simulink model "Simulink_Principal_Barbier_Touboul"  (R2020a)
settings: Solver=FixedStepAuto  StartTime=0.0  StopTime=fin  FixedStep=dt  RelTol=1e-4
values from neighbouring files (symbols this model uses):
  A = [teta1;teta2]    [visualisation_trame.m]
  Kd = 20*diag([1 1])    [visualisation_trame.m]
  Kp = 1e3*diag([1 1])    [visualisation_trame.m]
  P = 1e2*diag([1 1])    [visualisation_trame.m]
  S = 1e2*diag([1 1])    [visualisation_trame.m]
  Tau = [T1;T2]    [visualisation_trame.m]
undefined symbols (not defined in the file or in its folder): dyn, dyn2, dyn_mc_1, dyn_mc_2
settings Model: Creator=natha  LastModifiedBy=natha
settings DebuggingCC: ArithmeticOperatorsInVariantConditions=warning
settings SFSimCC: CustomCodeUndefinedFunction=UseInterfaceOnly

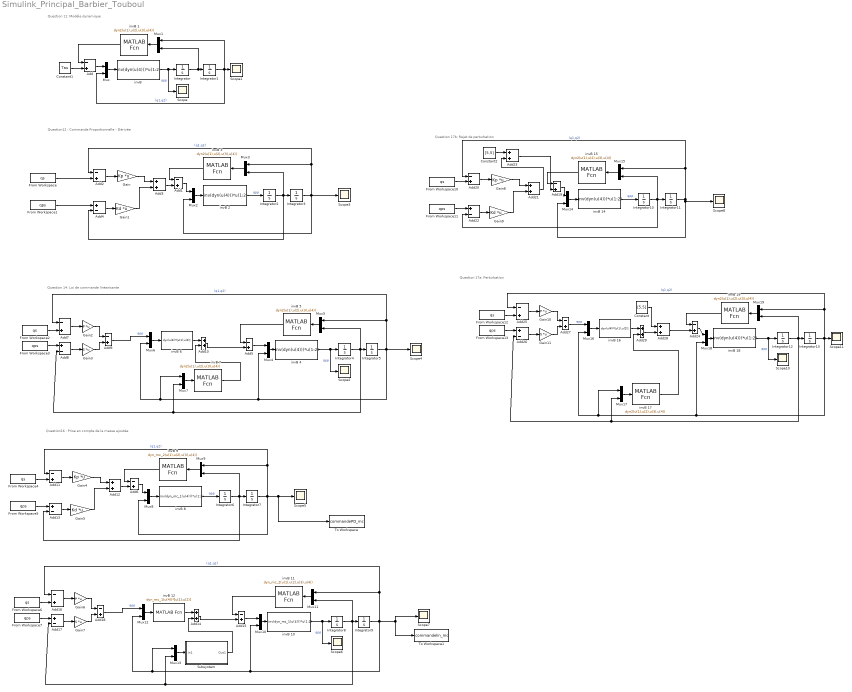
== system Simulink_Principal_Barbier_Touboul ==
  note: Question12 : Commande Proportionnelle - Dérivée
  note: Question 11: Modèle dynamique
  note: Question 14: Loi de commande linéarisante
  note: Question16 : Prise en compte de la masse ajoutée
  note: Question 17b: Rejet de perturbation
  note: Question 17a: Perturbation
  Add{,1..2,5..7,9,11,15..16,18..20,24..25,27} (16 alike) : Sum  Inputs=-+
  Add{3,10,12,14,21,23,28..29} (8 alike) : Sum
  Add{4,8,13,17,22,26} (6 alike) : Sum  Inputs=+-
  Constant : Constant  Value=[5,5]
  Constant1 : Constant  Value=Tau
  Constant2 : Constant  Value=[5,5]
  From Workspace{,2,4,6,10,12} (6 alike) : FromWorkspace  VariableName=qs
  From Workspace{1,3,5,7,11,13} (6 alike) : FromWorkspace  VariableName=qps
  Gain : Gain  Gain=Kp  Multiplication=Matrix(K*u)
  Gain1 : Gain  Gain=Kd  Multiplication=Matrix(K*u)
  Gain10 : Gain  Gain=P  Multiplication=Matrix(K*u)
  Gain11 : Gain  Gain=S  Multiplication=Matrix(K*u)
  Gain2 : Gain  Gain=P  Multiplication=Matrix(K*u)
  Gain3 : Gain  Gain=S  Multiplication=Matrix(K*u)
  Gain4 : Gain  Gain=Kp  Multiplication=Matrix(K*u)
  Gain5 : Gain  Gain=Kd  Multiplication=Matrix(K*u)
  Gain6 : Gain  Gain=P  Multiplication=Matrix(K*u)
  Gain7 : Gain  Gain=S  Multiplication=Matrix(K*u)
  Gain8 : Gain  Gain=Kp  Multiplication=Matrix(K*u)
  Gain9 : Gain  Gain=Kd  Multiplication=Matrix(K*u)
  Integrator{,1..2,4,6,8,10,12} (8 alike) : Integrator
  Integrator{3,5,7,9,11,13} (6 alike) : Integrator  InitialCondition=[A(1,1) A(2,1)]
  Mux{,1..19} (20 alike) : Mux  Inputs=2
  Scope{,1..8,10..11} (11 alike) : Scope
  Subsystem : Subsystem
  To Workspace : ToWorkspace  VariableName=commandePD_mc  SampleTime=-1
  To Workspace1 : ToWorkspace  VariableName=commandelin_mc  SampleTime=-1
  invB {,2,4,14,18} (5 alike) : MATLABFcn  MATLABFcn=inv(dyn(u(4)))*u(1:2)  OutputDimensions=2
      "invB " mask Display: disp('inv(M)*Tau')
      invB 14 mask Display: disp('inv(M)*Tau')
      invB 18 mask Display: disp('inv(M)*(Tau-H)')
      invB 2 mask Display: disp('inv(M)*Tau')
      invB 4 mask Display: disp('inv(M)*(Tau-H)')
  invB {1,3,5,7,15,17,19} (7 alike) : MATLABFcn  MATLABFcn=dyn2(u(1),u(2),u(3),u(4))  OutputDimensions=2
      mask Display: disp('H(q,qp)')
  invB 10 : MATLABFcn  MATLABFcn=inv(dyn_mc_1(u(4)))*u(1:2)  OutputDimensions=2
      mask Display: disp('inv(M)*(Tau-H)')
  invB 11 : MATLABFcn  MATLABFcn=dyn_mc_2(u(1),u(2),u(3),u(4))  OutputDimensions=2
      mask Display: disp('H(q,qp)')
  invB 12 : MATLABFcn  MATLABFcn=dyn_mc_1(u(4))*[u(1);u(2)]  OutputDimensions=2  Output1D=off
      mask Display: disp('M*(epp+qpps)')
  invB 16 : MATLABFcn  MATLABFcn=dyn(u(4))*[u(1);u(2)]  OutputDimensions=2  Output1D=off
      mask Display: disp('M*(epp+qpps)')
  invB 6 : MATLABFcn  MATLABFcn=dyn(u(4))*[u(1);u(2)]  OutputDimensions=2  Output1D=off
      mask Display: disp('M*(epp+qpps)')
  invB 8 : MATLABFcn  MATLABFcn=inv(dyn_mc_1(u(4)))*u(1:2)  OutputDimensions=2
      mask Display: disp('inv(M)*Tau')
  invB 9 : MATLABFcn  MATLABFcn=dyn_mc_2(u(1),u(2),u(3),u(4))  OutputDimensions=2
      mask Display: disp('H(q,qp)')
  wires:
  "invB "/1 -> Scope/1, Integrator/1  "qpp"
  Mux/1 -> "invB "/1
  Constant1/1 -> Add/2
  Integrator/1 -> Mux1/2, Integrator1/1
  Integrator1/1 -> Mux/2, Mux1/1, Scope1/1  "(q1,q2)"
  invB 1/1 -> Add/1
  Add/1 -> Mux/1
  Add1/1 -> Mux2/1
  Mux3/1 -> invB 3/1
  invB 2/1 -> Integrator2/1  "qpp"
  Mux2/1 -> invB 2/1
  invB 3/1 -> Add1/1
  Integrator2/1 -> Add4/2, Mux3/2, Integrator3/1
  Mux1/1 -> invB 1/1
  Add2/1 -> Gain/1
  Add3/1 -> Add1/2
  Gain/1 -> Add3/1
  Add4/1 -> Gain1/1
  Gain1/1 -> Add3/2
  Add10/1 -> Add5/2
  Mux5/1 -> invB 5/1
  invB 7/1 -> Add10/2
  Add9/1 -> Mux6/1  "epp"
  From Workspace2/1 -> Add7/2
  Integrator4/1 -> Add8/2, Mux7/2, Mux5/2, Integrator5/1
  Add7/1 -> Gain2/1
  Add8/1 -> Gain3/1
  Mux7/1 -> invB 7/1
  invB 6/1 -> Add10/1
  Mux4/1 -> invB 4/1
  invB 5/1 -> Add5/1
  Gain2/1 -> Add9/1
  Add5/1 -> Mux4/1
  Gain3/1 -> Add9/2
  invB 4/1 -> Integrator4/1, Scope2/1  "qpp"
  From Workspace3/1 -> Add8/1
  Mux6/1 -> invB 6/1
  From Workspace7/1 -> Add17/1
  Gain7/1 -> Add18/2
  Gain6/1 -> Add18/1
  Integrator9/1 -> Add16/1, Mux11/1, Mux10/2, Mux12/2, Mux13/1, Scope7/1, To Workspace1/1  "(q1,q2)"
  invB 10/1 -> Integrator8/1, Scope6/1  "qpp"
  Add15/1 -> Mux10/1
  invB 11/1 -> Add15/1
  Mux10/1 -> invB 10/1
  invB 12/1 -> Add14/1
  Add16/1 -> Gain6/1
  Mux12/1 -> invB 12/1
  Add17/1 -> Gain7/1
  Integrator8/1 -> Add17/2, Mux13/2, Mux11/2, Integrator9/1
  Add18/1 -> Mux12/1  "epp"
  From Workspace6/1 -> Add16/2
  Mux11/1 -> invB 11/1
  Add14/1 -> Add15/2
  From Workspace4/1 -> Add11/2
  From Workspace5/1 -> Add13/1
  Integrator6/1 -> Add13/2, Mux9/2, Integrator7/1
  Add11/1 -> Gain4/1
  Add13/1 -> Gain5/1
  Add6/1 -> Mux8/1
  invB 8/1 -> Integrator6/1  "qpp"
  Mux8/1 -> invB 8/1
  invB 9/1 -> Add6/1
  Mux9/1 -> invB 9/1
  Integrator7/1 -> Mux8/2, To Workspace/1, Scope5/1, Add11/1, Mux9/1  "(q1,q2)"
  Add12/1 -> Add6/2
  Gain5/1 -> Add12/2
  Gain4/1 -> Add12/1
  From Workspace/1 -> Add2/2
  From Workspace1/1 -> Add4/1
  Integrator10/1 -> Add22/2, Mux15/2, Integrator11/1
  Add23/1 -> Add19/2
  invB 14/1 -> Integrator10/1  "qpp"
  From Workspace10/1 -> Add20/2
  Gain9/1 -> Add21/2
  Mux14/1 -> invB 14/1
  Constant2/1 -> Add23/1
  Integrator3/1 -> Mux2/2, Scope3/1, Add2/1, Mux3/1  "(q1,q2)"
  Add19/1 -> Mux14/1
  Gain8/1 -> Add21/1
  Add22/1 -> Gain9/1
  Integrator11/1 -> Scope8/1, Mux14/2, Add20/1, Mux15/1  "(q1,q2)"
  Add20/1 -> Gain8/1
  Mux15/1 -> invB 15/1
  From Workspace11/1 -> Add22/1
  invB 15/1 -> Add19/1
  Add21/1 -> Add23/2
  From Workspace12/1 -> Add25/2
  Mux18/1 -> invB 18/1
  From Workspace13/1 -> Add26/1
  Integrator13/1 -> Mux16/2, Mux17/1, Mux18/2, Add25/1, Mux19/1, Scope11/1  "(q1,q2)"
  Gain10/1 -> Add27/1
  invB 18/1 -> Integrator12/1, Scope10/1  "qpp"
  Integrator5/1 -> Mux4/2, Mux6/2, Mux7/1, Scope4/1, Add7/1, Mux5/1  "(q1,q2)"
  Add27/1 -> Mux16/1  "epp"
  Constant/1 -> Add28/1
  Add25/1 -> Gain10/1
  invB 16/1 -> Add29/1
  Mux17/1 -> invB 17/1
  Add29/1 -> Add28/2
  Mux16/1 -> invB 16/1
  Add26/1 -> Gain11/1
  Integrator12/1 -> Add26/2, Mux17/2, Mux19/2, Integrator13/1
  invB 17/1 -> Add29/2
  Mux19/1 -> invB 19/1
  Add28/1 -> Add24/2
  Add24/1 -> Mux18/1
  invB 19/1 -> Add24/1
  Gain11/1 -> Add27/2
  Mux13/1 -> Subsystem/1(In1)
  Subsystem/1(Out1) -> Add14/2

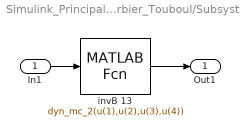
== system Simulink_Principal_Barbier_Touboul/Subsystem ==
  In1 : Inport
  invB 13 : MATLABFcn  MATLABFcn=dyn_mc_2(u(1),u(2),u(3),u(4))  OutputDimensions=2
      mask Display: disp('H(q,qp)')
  Out1 : Outport
  wires:
  In1/1 -> invB 13/1
  invB 13/1 -> Out1/1
